simulink model "4-2"  (R2021b)
settings: Solver=FixedStepDiscrete  StartTime=0.0  StopTime=10.0  RelTol=1e-3
undefined symbols (not defined in the file): sldvsubsys
libraries: simulink x5, sldvlib x4
settings Model: Creator=Alessandro  LastModifiedBy=Mattia
settings ConfigComp: DVMode=PropertyProving  DVTestSuiteOptimization=Auto  DVDetectOutOfBounds=on  DVModelReferenceHarness=on

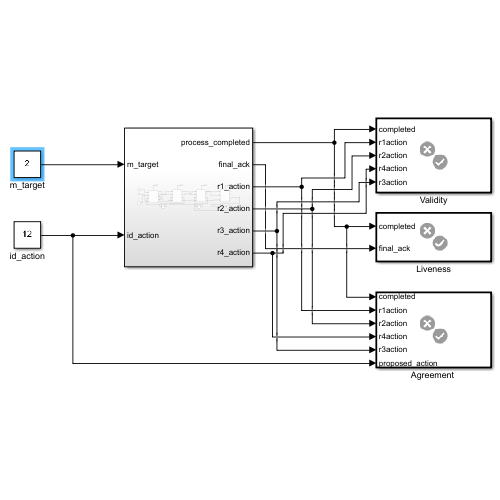
[thumbnail: Simulink's stored preview of the top-level diagram]
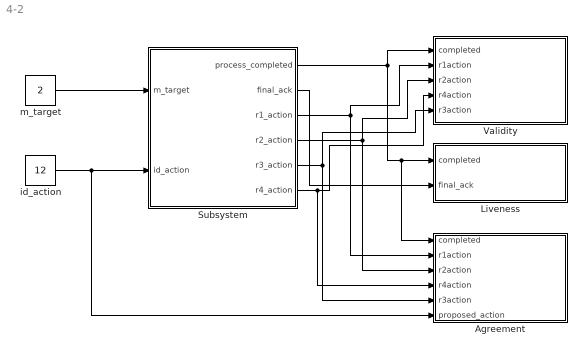
== system 4-2 ==
  "Agreement " : Subsystem  Tag=VerificationSubsystem  DisableCoverage=on  LoadFcn=sldvsubsys('check')  TreatAsAtomicUnit=on  SimViewingDevice=on  mask(VerificationSubsystem){}
      mask init:
      | sldvsubsys('maskInit');
      settings: CopyFcn=sldvsubsys('copy');  OpenFcn=open_system(gcb,'force');
      settings: PreSaveFcn=|
      | set_param(gcb,'SimViewingDevice','on');
      | sldvsubsys('check');
      mask Help: helpview(fullfile(docroot,'toolbox','sldv','sldv.map'),'verificationsubsystem')
      mask Display: image(imread('sldvicon_versubsys.png','BackGroundColor',[1 1 1]),'center');
  Liveness : Subsystem  Tag=VerificationSubsystem  DisableCoverage=on  LoadFcn=sldvsubsys('check')  TreatAsAtomicUnit=on  SimViewingDevice=on  mask(VerificationSubsystem){}
      mask init:
      | sldvsubsys('maskInit');
      settings: CopyFcn=sldvsubsys('copy');  OpenFcn=open_system(gcb,'force');
      settings: PreSaveFcn=|
      | set_param(gcb,'SimViewingDevice','on');
      | sldvsubsys('check');
      mask Help: helpview(fullfile(docroot,'toolbox','sldv','sldv.map'),'verificationsubsystem')
      mask Display: image(imread('sldvicon_versubsys.png','BackGroundColor',[1 1 1]),'center');
  Subsystem : Subsystem
  Validity : Subsystem  Tag=VerificationSubsystem  DisableCoverage=on  LoadFcn=sldvsubsys('check')  TreatAsAtomicUnit=on  SimViewingDevice=on  mask(VerificationSubsystem){}
      mask init:
      | sldvsubsys('maskInit');
      settings: CopyFcn=sldvsubsys('copy');  OpenFcn=open_system(gcb,'force');
      settings: PreSaveFcn=|
      | set_param(gcb,'SimViewingDevice','on');
      | sldvsubsys('check');
      mask Help: helpview(fullfile(docroot,'toolbox','sldv','sldv.map'),'verificationsubsystem')
      mask Display: image(imread('sldvicon_versubsys.png','BackGroundColor',[1 1 1]),'center');
  id_action : Constant  Value=12
  m_target : Constant  Value=2
  wires:
  m_target/1 -> Subsystem/1(m_target)
  id_action/1 -> "Agreement "/6(proposed_action), Subsystem/2(id_action)
  Subsystem/1(process_completed) -> Validity/1(completed), Liveness/1(completed), "Agreement "/1(completed)
  Subsystem/2(final_ack) -> Liveness/2(final_ack)
  Subsystem/3(r1_action) -> Validity/2(r1action), "Agreement "/2(r1action)
  Subsystem/4(r2_action) -> Validity/3(r2action), "Agreement "/3(r2action)
  Subsystem/5(r3_action) -> "Agreement "/5(r3action), Validity/5(r3action)
  Subsystem/6(r4_action) -> "Agreement "/4(r4action), Validity/4(r4action)

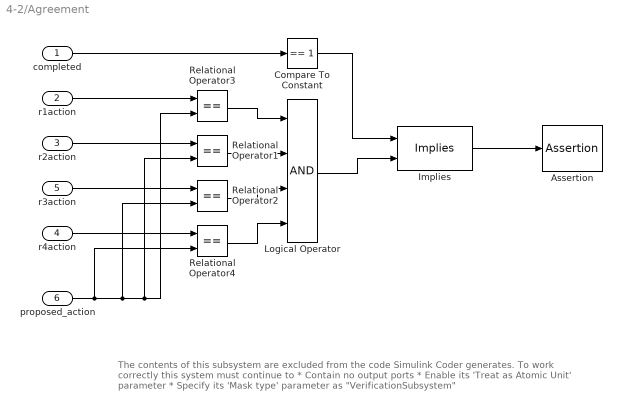
== system 4-2/Agreement  ==
  note: The contents of this subsystem are excluded from the code Simulink Coder
      | generates.
      |
      | To work correctly this system must continue to
      | * Contain no output ports
      | * Enable its 'Treat as Atomic Unit' parameter
      | * Specify its 'Mask type' parameter as "VerificationSubsystem"
  completed : Inport
  r1action : Inport  Port=2
  r2action : Inport  Port=3
  r4action : Inport  Port=4
  r3action : Inport  Port=5
  proposed_action : Inport  Port=6
  Assertion : Assertion  StopWhenAssertionFail=off
  Compare To Constant : simulink/Logic and Bit Operations/Compare To Constant  relop===  const=1  OutDataTypeStr=boolean
  Implies : sldvlib/Verification Utilities/Implies
      settings: SourceProductBaseCode=SL
  Logical Operator : Logic  Inputs=4  AllPortsSameDT=off  OutDataTypeStr=boolean
  Relational Operator{1..4} (4 alike) : RelationalOperator  Operator===  OutDataTypeStr=boolean  RndMeth=Simplest
  wires:
  completed/1 -> Compare To Constant/1
  Compare To Constant/1 -> Implies/1
  Logical Operator/1 -> Implies/2
  Implies/1 -> Assertion/1
  r1action/1 -> Relational Operator3/1
  r2action/1 -> Relational Operator1/1
  r3action/1 -> Relational Operator2/1
  r4action/1 -> Relational Operator4/1
  proposed_action/1 -> Relational Operator4/2, Relational Operator2/2, Relational Operator1/2, Relational Operator3/2
  Relational Operator3/1 -> Logical Operator/1
  Relational Operator1/1 -> Logical Operator/2
  Relational Operator2/1 -> Logical Operator/3
  Relational Operator4/1 -> Logical Operator/4

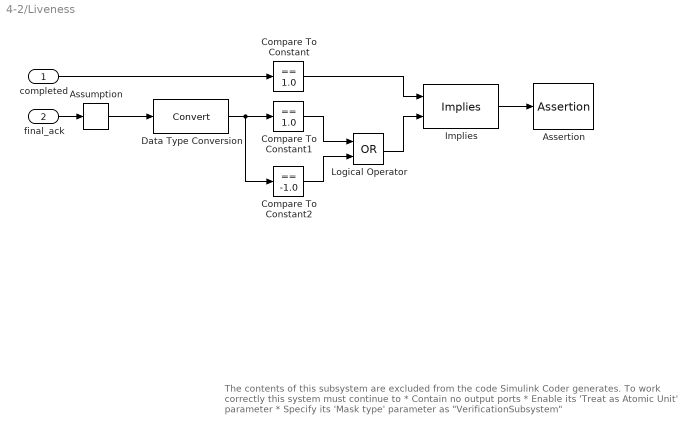
== system 4-2/Liveness ==
  note: The contents of this subsystem are excluded from the code Simulink Coder
      | generates.
      |
      | To work correctly this system must continue to
      | * Contain no output ports
      | * Enable its 'Treat as Atomic Unit' parameter
      | * Specify its 'Mask type' parameter as "VerificationSubsystem"
  completed : Inport
  final_ack : Inport  Port=2
  Assertion : Assertion
  Assumption : sldvlib/Objectives and Constraints/Assumption  enabled=on  customAVTBlockType=Assumption  intervals={-1,1}  initial=off  dispValues=on  outEnabled=on
      settings: AttributesFormatString=%<intervals>  SourceProductBaseCode=SL
  Compare To Constant : simulink/Logic and Bit Operations/Compare To Constant  relop===  const=1.0  OutDataTypeStr=boolean
  Compare To Constant1 : simulink/Logic and Bit Operations/Compare To Constant  relop===  const=1.0  OutDataTypeStr=boolean
  Compare To Constant2 : simulink/Logic and Bit Operations/Compare To Constant  relop===  const=-1.0  OutDataTypeStr=boolean
  Data Type Conversion : DataTypeConversion
  Implies : sldvlib/Verification Utilities/Implies
      settings: SourceProductBaseCode=SL
  Logical Operator : Logic  Operator=OR  AllPortsSameDT=off  OutDataTypeStr=boolean
  wires:
  completed/1 -> Compare To Constant/1
  Compare To Constant1/1 -> Logical Operator/1
  Compare To Constant2/1 -> Logical Operator/2
  Compare To Constant/1 -> Implies/1
  Logical Operator/1 -> Implies/2
  Implies/1 -> Assertion/1
  final_ack/1 -> Assumption/1
  Assumption/1 -> Data Type Conversion/1
  Data Type Conversion/1 -> Compare To Constant2/1, Compare To Constant1/1

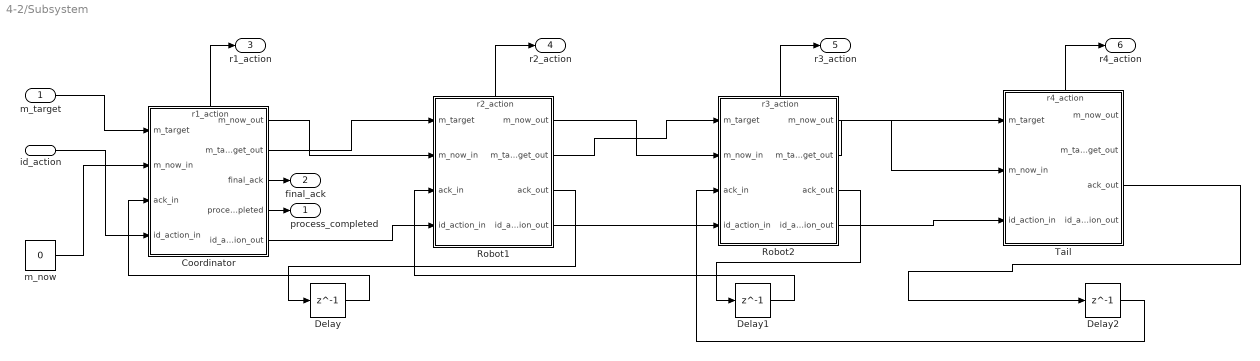
== system 4-2/Subsystem ==
  m_target : Inport
  id_action : Inport  Port=2
  Coordinator : Stateflow chart  TreatAsAtomicUnit=on
      settings: PortSchema="{\"entries\":[{\"content\":{\"sides\":[{\"content\":{\"connectorIds\":[\"In1\",\"In2\",\"In3\",\"In4\"]},\"type\":\"ConnectorPlacement.EquallySpacedRectSide\",\"uuid\":\"f207236c-0599-4b46-9b3f-c0f809d9e1de\"},{\"content\":{\"connectorIds\":[\"Out2\",\"Out3\",\"Out4\",\"Out5\",\"Out6\"],\"side\":\"RIGHT\"},\"type\":\"ConnectorPlacement.EquallySpacedRectSide\",\"uuid\":\"63272974-e9ab-41b4-a3ca-cff66dd5b970\"},{\"content\":{\"connectorIds\":[\"Out1\"],\"side\":\"TOP\"},\"type\":\"ConnectorPlacement.EquallySpacedRectSide\",\"uuid\":\"6ce3df78-5d10-4d9a-bb6f-21eee9393606\"}]},\"type\":\"ConnectorPlacement.EquallySpacedConnector\",\"uuid\":\"1a0d068b-3bbf-4b25-a405-60ce12d31816\"}],\"packageUris\":[\"http://schema.mathworks.com/mf0/Connector/R2020b\"],\"version\":\"1.0\"}"
  Delay : Delay  DelayLength=1  InitialCondition=0
  Delay1 : Delay  DelayLength=1  InitialCondition=0
  Delay2 : Delay  DelayLength=1  InitialCondition=0
  Robot1 : Stateflow chart  TreatAsAtomicUnit=on
      settings: PortSchema="{\"entries\":[{\"content\":{\"sides\":[{\"content\":{\"connectorIds\":[\"In1\",\"In2\",\"In3\",\"In4\"]},\"type\":\"ConnectorPlacement.EquallySpacedRectSide\",\"uuid\":\"0bb30c5a-43df-4072-a77c-4a1dce14f9fe\"},{\"content\":{\"connectorIds\":[\"Out2\",\"Out3\",\"Out4\",\"Out5\"],\"side\":\"RIGHT\"},\"type\":\"ConnectorPlacement.EquallySpacedRectSide\",\"uuid\":\"e534c186-56c2-4af4-b3f1-02d020398bac\"},{\"content\":{\"connectorIds\":[\"Out1\"],\"side\":\"TOP\"},\"type\":\"ConnectorPlacement.EquallySpacedRectSide\",\"uuid\":\"e2ef603c-6980-4fc1-bc1c-88b0ffffdb44\"}]},\"type\":\"ConnectorPlacement.EquallySpacedConnector\",\"uuid\":\"7e88c6c9-7de7-4b98-93fa-510699497ff0\"}],\"packageUris\":[\"http://schema.mathworks.com/mf0/Connector/R2020b\"],\"version\":\"1.0\"}"
  Robot2 : Stateflow chart  TreatAsAtomicUnit=on
      settings: PortSchema="{\"entries\":[{\"content\":{\"sides\":[{\"content\":{\"connectorIds\":[\"In1\",\"In2\",\"In3\",\"In4\"]},\"type\":\"ConnectorPlacement.EquallySpacedRectSide\",\"uuid\":\"0bb30c5a-43df-4072-a77c-4a1dce14f9fe\"},{\"content\":{\"connectorIds\":[\"Out2\",\"Out3\",\"Out4\",\"Out5\"],\"side\":\"RIGHT\"},\"type\":\"ConnectorPlacement.EquallySpacedRectSide\",\"uuid\":\"e534c186-56c2-4af4-b3f1-02d020398bac\"},{\"content\":{\"connectorIds\":[\"Out1\"],\"side\":\"TOP\"},\"type\":\"ConnectorPlacement.EquallySpacedRectSide\",\"uuid\":\"e2ef603c-6980-4fc1-bc1c-88b0ffffdb44\"}]},\"type\":\"ConnectorPlacement.EquallySpacedConnector\",\"uuid\":\"7e88c6c9-7de7-4b98-93fa-510699497ff0\"}],\"packageUris\":[\"http://schema.mathworks.com/mf0/Connector/R2020b\"],\"version\":\"1.0\"}"
  Tail : Stateflow chart  TreatAsAtomicUnit=on
      settings: PortSchema="{\"entries\":[{\"content\":{\"sides\":[{\"content\":{\"connectorIds\":[\"In1\",\"In2\",\"In3\"]},\"type\":\"ConnectorPlacement.EquallySpacedRectSide\",\"uuid\":\"8f0c7a78-6297-425d-9fc8-91e71c821e74\"},{\"content\":{\"connectorIds\":[\"Out2\",\"Out3\",\"Out4\",\"Out5\"],\"side\":\"RIGHT\"},\"type\":\"ConnectorPlacement.EquallySpacedRectSide\",\"uuid\":\"2a4e4ba2-0ea2-4b66-9720-65f8c6802208\"},{\"content\":{\"connectorIds\":[\"Out1\"],\"side\":\"TOP\"},\"type\":\"ConnectorPlacement.EquallySpacedRectSide\",\"uuid\":\"3c4e4337-d1ab-4209-abe4-e09ccc9a45b1\"}]},\"type\":\"ConnectorPlacement.EquallySpacedConnector\",\"uuid\":\"5f75d573-6dad-4549-ba0d-242a5d54a9e5\"}],\"packageUris\":[\"http://schema.mathworks.com/mf0/Connector/R2020b\"],\"version\":\"1.0\"}"
  m_now : Constant  Value=0
  process_completed : Outport
  final_ack : Outport  Port=2
  r1_action : Outport  Port=3
  r2_action : Outport  Port=4
  r3_action : Outport  Port=5
  r4_action : Outport  Port=6
  wires:
  m_now/1 -> Coordinator/2(m_now_in)
  m_target/1 -> Coordinator/1(m_target)
  Delay/1 -> Coordinator/3(ack_in)
  Coordinator/2(m_now_out) -> Robot1/2(m_now_in)
  Coordinator/3(m_target_out) -> Robot1/1(m_target)
  Robot1/4(ack_out) -> Delay/1
  Coordinator/5(process_completed) -> process_completed/1
  Coordinator/4(final_ack) -> final_ack/1
  id_action/1 -> Coordinator/4(id_action_in)
  Coordinator/6(id_action_out) -> Robot1/4(id_action_in)
  Robot1/2(m_now_out) -> Robot2/2(m_now_in)
  Robot1/3(m_target_out) -> Robot2/1(m_target)
  Robot1/5(id_action_out) -> Robot2/4(id_action_in)
  Robot2/2(m_now_out) -> Tail/2(m_now_in)
  Robot2/3(m_target_out) -> Tail/1(m_target)
  Robot2/5(id_action_out) -> Tail/3(id_action_in)
  Robot2/4(ack_out) -> Delay1/1
  Delay1/1 -> Robot1/3(ack_in)
  Tail/4(ack_out) -> Delay2/1
  Delay2/1 -> Robot2/3(ack_in)
  Coordinator/1(r1_action) -> r1_action/1
  Robot1/1(r2_action) -> r2_action/1
  Robot2/1(r3_action) -> r3_action/1
  Tail/1(r4_action) -> r4_action/1

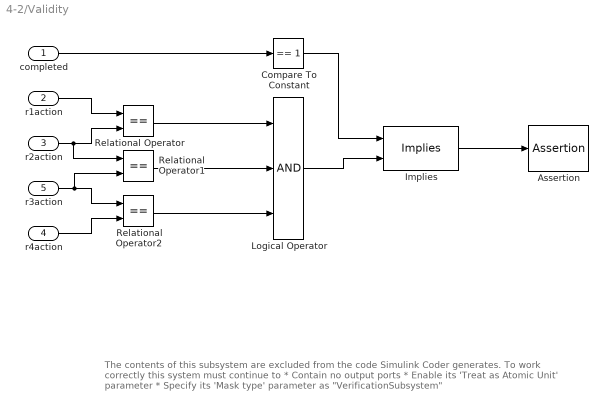
== system 4-2/Validity ==
  note: The contents of this subsystem are excluded from the code Simulink Coder
      | generates.
      |
      | To work correctly this system must continue to
      | * Contain no output ports
      | * Enable its 'Treat as Atomic Unit' parameter
      | * Specify its 'Mask type' parameter as "VerificationSubsystem"
  completed : Inport
  r1action : Inport  Port=2
  r2action : Inport  Port=3
  r4action : Inport  Port=4
  r3action : Inport  Port=5
  Assertion : Assertion  StopWhenAssertionFail=off
  Compare To Constant : simulink/Logic and Bit Operations/Compare To Constant  relop===  const=1  OutDataTypeStr=boolean
  Implies : sldvlib/Verification Utilities/Implies
      settings: SourceProductBaseCode=SL
  Logical Operator : Logic  Inputs=3  AllPortsSameDT=off  OutDataTypeStr=boolean
  Relational Operator : RelationalOperator  Operator===  OutDataTypeStr=boolean  RndMeth=Simplest
  Relational Operator1 : RelationalOperator  Operator===  OutDataTypeStr=boolean  RndMeth=Simplest
  Relational Operator2 : RelationalOperator  Operator===  OutDataTypeStr=boolean  RndMeth=Simplest
  wires:
  completed/1 -> Compare To Constant/1
  Relational Operator/1 -> Logical Operator/1
  Relational Operator1/1 -> Logical Operator/2
  Relational Operator2/1 -> Logical Operator/3
  Compare To Constant/1 -> Implies/1
  Logical Operator/1 -> Implies/2
  Implies/1 -> Assertion/1
  r1action/1 -> Relational Operator/1
  r2action/1 -> Relational Operator1/1, Relational Operator/2
  r3action/1 -> Relational Operator1/2, Relational Operator2/1
  r4action/1 -> Relational Operator2/2

== stateflow chart 4-2/Subsystem/Robot1 ==
  state FeedForward
    entry:
    r2_action = id_action_in;
    m_target_out = m_target
    id_action_out = id_action_in;
  state Initial
    entry:
    gen = 0;
    if gen>0.5
    m_now_out = m_now_in + 1;
    end
  state EnoughRobots1
    entry:
    r2_action = id_action_in;
    ack_out = ack_in;
  (default) -> Initial
  Initial -> FeedForward
  FeedForward -> EnoughRobots1 : [ack_in == 1 || ack_in == -1]
  data: r function_output; r2_action output; m_target input; m_now_in input; m_now_out output; gen local; m_target_out output; ack_in input; ack_out output; id_action_in input; id_action_out output
  function r = Random:
    | function r = Random
    | %#codegen
    | rng(2);
    | r = rand(1);
    | end

== stateflow chart 4-2/Subsystem/Tail ==
  state FeedForward
    entry:
    ack_out  = 1;
    r4_action = id_action_in;
  state Initial
    entry:
    r4_action = id_action_in;
    id_action_out = id_action_in;
    gen = Random();
    if gen>0.5
    m_now_out = m_now_in + 1;
    else
    m_now_out = m_now_in;
    end
  state EnoughRobots
    entry:
    ack_out  = -1;
    r4_action = id_action_in;
    m_target_out = m_target;
  (default) -> Initial
  Initial -> FeedForward [order 2] : [m_now_out >= m_target]
  Initial -> EnoughRobots [order 1] : [m_now_out < m_target]
  data: r function_output; r4_action output; m_target input; m_now_in input; m_now_out output; gen local; m_target_out output; ack_out output; id_action_in input; id_action_out output
  function r = Random:
    | function r = Random
    | %#codegen
    | rng(4);
    | r = rand(1);
    | end

== stateflow chart 4-2/Subsystem/Coordinator ==
  state FeedForward
    entry:
    m_target_out = m_target
    id_action_out = id_action_in;
  state Initial
    entry:
    r1_action = id_action_in;
    gen = Random();
    if gen>0.5
    m_now_out = m_now_in + 1;
    end
  state EnoughRobots1
    process_completed=1;
    final_ack = ack_in;
  (default) -> Initial
  Initial -> FeedForward
  FeedForward -> EnoughRobots1 : [ack_in == 1 || ack_in == -1]
  data: r function_output; r1_action output; m_target input; m_now_in input; m_now_out output; gen local; m_target_out output; ack_in input; final_ack output; process_completed output; id_action_in input; id_action_out output
  function r = Random:
    | function r = Random
    | %#codegen
    | rng(1);
    | r = rand(1);
    | end

== stateflow chart 4-2/Subsystem/Robot2 ==
  state FeedForward
    entry:
    m_target_out = m_target
    id_action_out = id_action_in;
    r3_action = id_action_in;
  state Initial
    entry:
    r3_action = id_action_in;
    gen = 0;
    if gen>0.5
    m_now_out = m_now_in + 1;
    end
  state EnoughRobots1
    entry:
    ack_out = ack_in;
    r3_action = id_action_in;
  (default) -> Initial
  Initial -> FeedForward
  FeedForward -> EnoughRobots1 : [ack_in == 1 || ack_in == -1]
  data: r function_output; r3_action output; m_target input; m_now_in input; m_now_out output; gen local; m_target_out output; ack_in input; ack_out output; id_action_in input; id_action_out output
  function r = Random:
    | function r = Random
    | %#codegen
    | rng(3);
    | r = rand(1);
    | end
